simulink model "kundur_cvs_p1"  (R2025b)
settings: Solver=ode23t  StartTime=0.0  StopTime=0.5  MaxStep=0.005  RelTol=1e-3
libraries: spsGroundLib x5, spsSeriesRLCBranchLib x5, spsControlledVoltageSourceLib x4, spsACVoltageSourceLib x1, spspowerguiLib x1
settings Model: Creator=27443  LastModifiedBy=27443

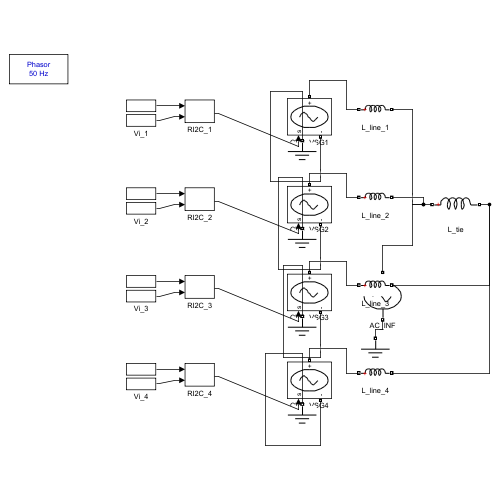
[thumbnail: Simulink's stored preview of the top-level diagram]
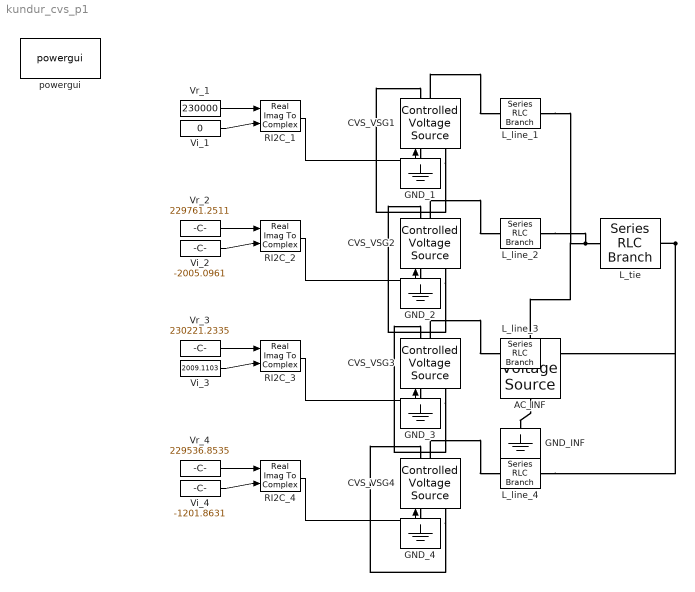
== system kundur_cvs_p1 ==
  AC_INF : spsACVoltageSourceLib/AC Voltage Source  Amplitude=230000  Phase=0  Frequency=50  SampleTime=0  Measurements=None  BusType=swing  Pref=10e3  Qref=0  Qmin=-inf  Qmax=+inf
  CVS_VSG{1..4} (4 alike) : spsControlledVoltageSourceLib/Controlled Voltage Source  Initialize=off  Source_Type=DC  Amplitude=230000  Phase=0  Frequency=0  Measurements=None
  GND_{1..4} (4 alike) : spsGroundLib/Ground  LConnTagsString=a
  GND_INF : spsGroundLib/Ground  LConnTagsString=a
  L_line_{1..4} (4 alike) : spsSeriesRLCBranchLib/Series RLC Branch  LConnTagsString=__new0  RConnTagsString=__new0  BranchType=L  Resistance=1  Inductance=0.16839  SetiL0=off  InitialCurrent=0  Capacitance=1e-6  Setx0=off  InitialVoltage=0  Measurements=None
  L_tie : spsSeriesRLCBranchLib/Series RLC Branch  LConnTagsString=__new0  RConnTagsString=__new0  BranchType=L  Resistance=1  Inductance=0.50516  SetiL0=off  InitialCurrent=0  Capacitance=1e-6  Setx0=off  InitialVoltage=0  Measurements=None
  RI2C_{1..4} (4 alike) : RealImagToComplex
  Vi_1 : Constant  Value=0
  Vi_2 : Constant  Value=-2005.0961
  Vi_3 : Constant  Value=2009.1103
  Vi_4 : Constant  Value=-1201.8631
  Vr_1 : Constant  Value=230000
  Vr_2 : Constant  Value=229761.2511
  Vr_3 : Constant  Value=230221.2335
  Vr_4 : Constant  Value=229536.8535
  powergui : spspowerguiLib/powergui  Priority=1  SimulationMode=Phasor  SampleTime=50e-6  frequency=50  Iterations=50  frequencyindice=60  Pbase=100e6  ErrMax=1e-4  UnitsV=kV  UnitsW=MW  buscounter=0  FunctionMessages=off  echomessages=off  EnableUseOfTLC=off  CurrentSourceSwitches=off  DisableSnubberDevices=off  DisableRonSwitches=off  DisableVfSwitches=off  DisplayEquations=off  AutomaticDiscreteSolvers=off  SolverType=Tustin/Backward Euler (TBE)  Interpol=off  ExternalGateDelay=off  methode=off  Ts=100  x0status=blocks  SPID=on  SwTol=0  HookPort=off  NonlinearTolerance=1e-4  nMaxIteration=100  ContinueOnMaxIteration=off  RestoreLinks=warning  ResistiveCurrentMeasurement=off  Frange=[0:2:500]  Ylog=off  Xlog=on  ShowGrid=off  save=off  variable=ZData  structure=0  ZoomFFT=off  StartTime=0.0  cycles=1  DisplayStyle=1  fundamental=60  FreqAxis=off  MaxFrequency=1000  frequencyindicesteady=1  RmsSteady=1  display=off
  wires:
  Vr_1/1 -> RI2C_1/1
  Vi_1/1 -> RI2C_1/2
  RI2C_1/1 -> CVS_VSG1/1
  Vr_2/1 -> RI2C_2/1
  Vi_2/1 -> RI2C_2/2
  RI2C_2/1 -> CVS_VSG2/1
  Vr_3/1 -> RI2C_3/1
  Vi_3/1 -> RI2C_3/2
  RI2C_3/1 -> CVS_VSG3/1
  Vr_4/1 -> RI2C_4/1
  Vi_4/1 -> RI2C_4/2
  RI2C_4/1 -> CVS_VSG4/1
  connections:
  CVS_VSG1/RConn1 -- L_line_1/LConn1
  L_line_1/RConn1 -- L_line_2/RConn1 -- L_tie/LConn1 -- AC_INF/RConn1
  CVS_VSG1/LConn1 -- GND_1/LConn1
  CVS_VSG2/RConn1 -- L_line_2/LConn1
  CVS_VSG2/LConn1 -- GND_2/LConn1
  CVS_VSG3/RConn1 -- L_line_3/LConn1
  L_tie/RConn1 -- L_line_3/RConn1 -- L_line_4/RConn1
  CVS_VSG3/LConn1 -- GND_3/LConn1
  CVS_VSG4/RConn1 -- L_line_4/LConn1
  CVS_VSG4/LConn1 -- GND_4/LConn1
  AC_INF/LConn1 -- GND_INF/LConn1
